simulink library "rotationFromGroundToTangent"  (R2020a)
settings: Solver=VariableStepAuto  StartTime=0.0  StopTime=10.0  RelTol=1e-3
libraries: rotationAboutZ x2, rotationAboutY x1
settings Model: Creator=Ayaz  LastModifiedBy=Ayaz

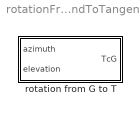
== system rotationFromGroundToTangent ==
  rotation from G to T : Subsystem

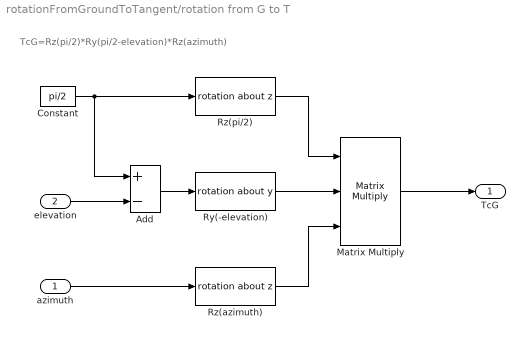
== system rotationFromGroundToTangent/rotation from G to T ==
  note: TcG=Rz(pi/2)*Ry(pi/2-elevation)*Rz(azimuth)
  azimuth : Inport
  elevation : Inport  Port=2
  Add : Sum  Inputs=+-
  Constant : Constant  Value=pi/2  VectorParams1D=off
  Matrix Multiply : Product  Inputs=3  Multiplication=Matrix(*)
  Ry(-elevation) : rotationAboutY/rotation about y  SystemSampleTime=-1  Latency=0  AutoFrameSizeCalculation=off
  Rz(azimuth) : rotationAboutZ/rotation about z  SystemSampleTime=-1  Latency=0  AutoFrameSizeCalculation=off
  Rz(pi/2) : rotationAboutZ/rotation about z  SystemSampleTime=-1  Latency=0  AutoFrameSizeCalculation=off
  TcG : Outport
  wires:
  azimuth/1 -> Rz(azimuth)/1
  elevation/1 -> Add/2
  Add/1 -> Ry(-elevation)/1
  Constant/1 -> Add/1, Rz(pi/2)/1
  Rz(pi/2)/1 -> Matrix Multiply/1
  Ry(-elevation)/1 -> Matrix Multiply/2
  Rz(azimuth)/1 -> Matrix Multiply/3
  Matrix Multiply/1 -> TcG/1
